simulink model "a0427"  (R2018b)
settings: Solver=VariableStepAuto  StartTime=0.0  StopTime=120  RelTol=1e-3
libraries: simulink x2
settings Model: Creator=chpark  LastModifiedBy=chpark

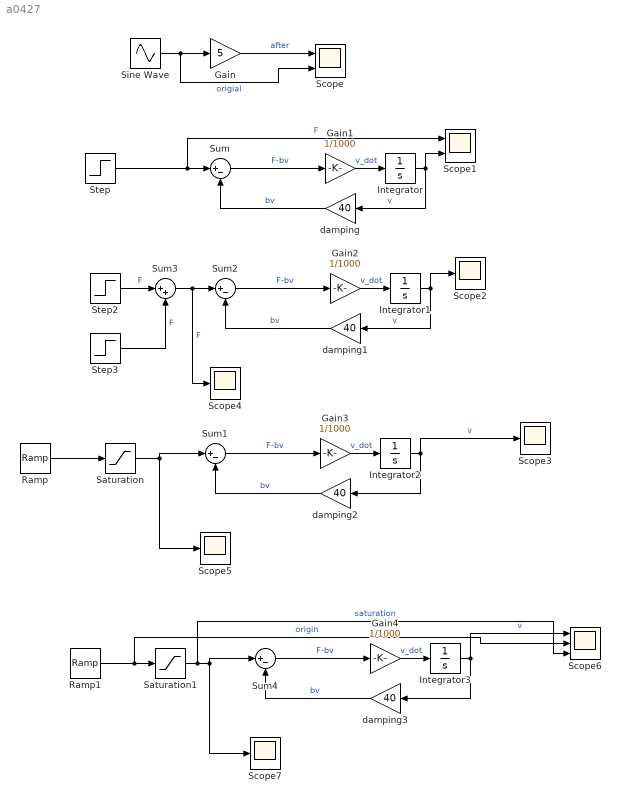
== system a0427 ==
  Gain : Gain  Gain=5
  Gain{1..4} (4 alike) : Gain  Gain=1/1000
  Integrator{,1..3} (4 alike) : Integrator
  Ramp : simulink/Sources/Ramp  slope=80  start=0  InitialOutput=0
  Ramp1 : simulink/Sources/Ramp  slope=80  start=0  InitialOutput=0
  Saturation : Saturate  UpperLimit=2000
  Saturation1 : Saturate  UpperLimit=2000
  Scope : Scope  NumInputPorts=2
  Scope1 : Scope  NumInputPorts=2
  Scope{2..5,7} (5 alike) : Scope
  Scope6 : Scope  NumInputPorts=3
  Sine Wave : Sin  Amplitude=2  Frequency=pi  Phase=pi/2  SampleTime=0
  Step : Step  Time=0  After=400  SampleTime=0
  Step2 : Step  Time=100  After=-400  SampleTime=0
  Step3 : Step  Time=0  After=400  SampleTime=0
  Sum{,1..2,4} (4 alike) : Sum  Inputs=|+-
  Sum3 : Sum  Inputs=|++
  damping{,1..3} (4 alike) : Gain  Gain=40
  wires:
  Sum/1 -> Gain1/1  "F-bv"
  Integrator/1 -> damping/1, Scope1/2  "v"
  Gain1/1 -> Integrator/1  "v_dot"
  damping/1 -> Sum/2  "bv"
  Sine Wave/1 -> Scope/2, Gain/1  "origial"
  Gain/1 -> Scope/1  "after"
  Step/1 -> Scope1/1, Sum/1  "F"
  damping1/1 -> Sum2/2  "bv"
  Gain2/1 -> Integrator1/1  "v_dot"
  Step2/1 -> Sum3/1  "F"
  Sum2/1 -> Gain2/1  "F-bv"
  Step3/1 -> Sum3/2  "F"
  Integrator1/1 -> Scope2/1, damping1/1  "v"
  Sum3/1 -> Scope4/1, Sum2/1  "F"
  Integrator2/1 -> Scope3/1, damping2/1  "v"
  Sum1/1 -> Gain3/1  "F-bv"
  damping2/1 -> Sum1/2  "bv"
  Gain3/1 -> Integrator2/1  "v_dot"
  Ramp/1 -> Saturation/1
  Saturation/1 -> Sum1/1, Scope5/1
  Ramp1/1 -> Scope6/2, Saturation1/1  "origin"
  Saturation1/1 -> Scope6/3, Sum4/1, Scope7/1  "saturation"
  Integrator3/1 -> Scope6/1, damping3/1  "v"
  Gain4/1 -> Integrator3/1  "v_dot"
  damping3/1 -> Sum4/2  "bv"
  Sum4/1 -> Gain4/1  "F-bv"
